simulink model "control"  (R2019a)
settings: Solver=VariableStepAuto  StartTime=0.0  StopTime=1500  RelTol=1e-3
settings Model: Creator=josefernandorosaribeiro  LastModifiedBy=josefernandorosaribeiro

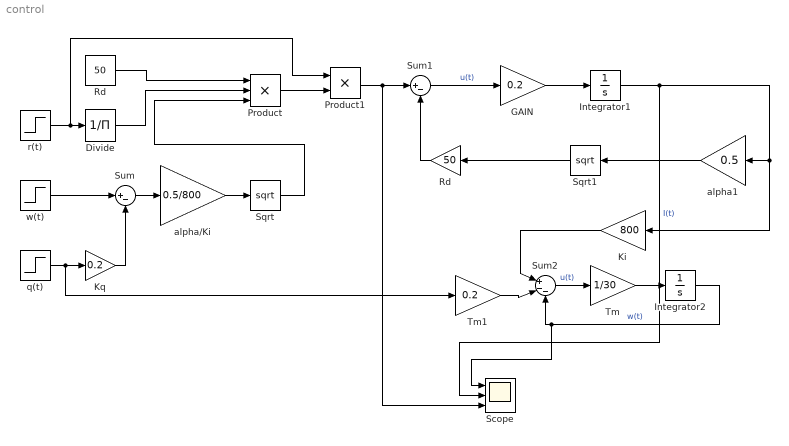
== system control ==
  Divide : Product  Inputs=/
  GAIN : Gain  Gain=0.2
  Integrator1 : Integrator
  Integrator2 : Integrator  InitialCondition=15
  Ki : Gain  Gain=800
  Kq : Gain  Gain=0.2
  Product : Product  Inputs=3
  Product1 : Product
  Rd : Gain  Gain=50
  "Rd " : Constant  Value=50
  Scope : Scope  NumInputPorts=3
  Sqrt : Sqrt  SaturateOnIntegerOverflow=on
  Sqrt1 : Sqrt  SaturateOnIntegerOverflow=on
  Sum : Sum  Inputs=|+-
  Sum1 : Sum  Inputs=|+-
  Sum2 : Sum  Inputs=|+--
  Tm : Gain  Gain=1/30
  Tm1 : Gain  Gain=0.2
  alpha/Ki : Gain  Gain=0.5/800
  alpha1 : Gain  Gain=0.5
  q(t) : Step  SampleTime=0
  r(t) : Step  Before=1  SampleTime=0
  w(t) : Step  Before=1  SampleTime=0
  wires:
  r(t)/1 -> Product1/1, Divide/1
  Divide/1 -> Product/2
  "Rd "/1 -> Product/1
  w(t)/1 -> Sum/1
  Kq/1 -> Sum/2
  Sum/1 -> alpha/Ki/1
  alpha/Ki/1 -> Sqrt/1
  Sqrt/1 -> Product/3
  Product/1 -> Product1/2
  Sqrt1/1 -> Rd/1
  GAIN/1 -> Integrator1/1
  Sum1/1 -> GAIN/1  "u(t)"
  alpha1/1 -> Sqrt1/1
  q(t)/1 -> Tm1/1, Kq/1
  Ki/1 -> Sum2/1
  Integrator2/1 -> Scope/1, Sum2/3  "w(t)"
  Rd/1 -> Sum1/2
  Sum2/1 -> Tm/1  "u(t)"
  Tm1/1 -> Sum2/2
  Integrator1/1 -> Scope/2, Ki/1, alpha1/1  "I(t)"
  Tm/1 -> Integrator2/1
  Product1/1 -> Scope/3, Sum1/1
